simulink model "Simulation"  (R2021a)
settings: Solver=VariableStepAuto  StartTime=0.0  StopTime=10.0  RelTol=1e-3
undefined symbols (not defined in the file or in its folder): Gp_Den, Gp_Num, Ts
settings Model: Creator=arman  LastModifiedBy=arman

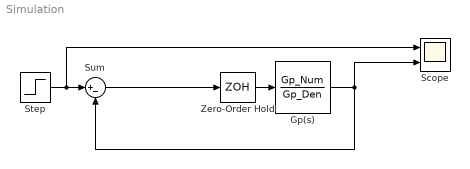
== system Simulation ==
  Gp(s) : TransferFcn  Numerator=Gp_Num  Denominator=Gp_Den
  Scope : Scope  NumInputPorts=2
  Step : Step  SampleTime=0
  Sum : Sum  Inputs=|+-
  Zero-Order Hold : ZeroOrderHold  SampleTime=Ts
  wires:
  Zero-Order Hold/1 -> Gp(s)/1
  Gp(s)/1 -> Sum/2, Scope/2
  Step/1 -> Scope/1, Sum/1
  Sum/1 -> Zero-Order Hold/1
